simulink model "M182_Lab2"  (R2019b)
settings: Solver=ode45  StartTime=0.0  StopTime=10  RelTol=1e-5
settings Model: Creator=scjcb  LastModifiedBy=scjcb

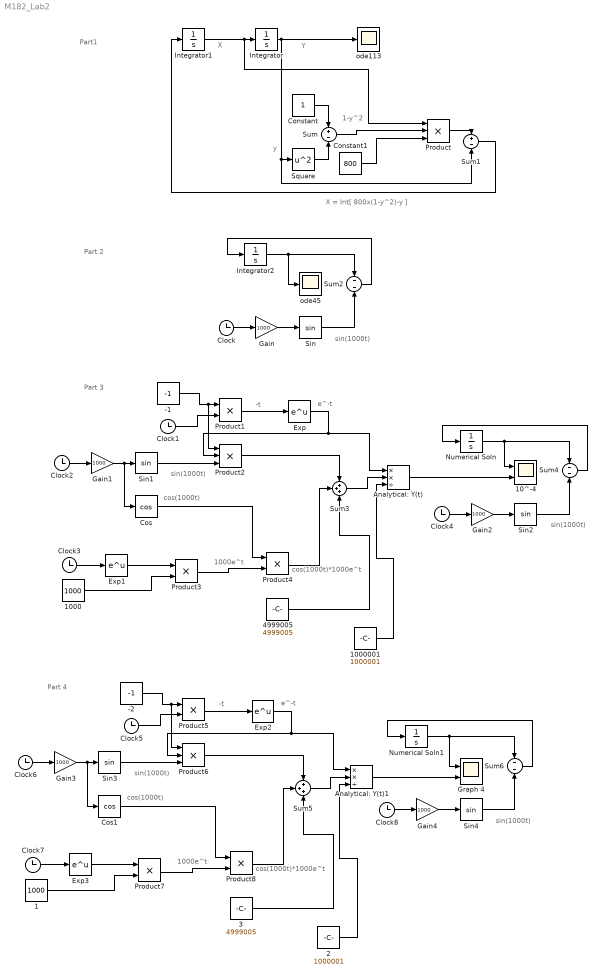
== system M182_Lab2 ==
  note: Part 3
  note: Part 2
  note: Part1
  note: cos(1000t)*1000e^t
  note: cos(1000t)
  note: 1000e^t
  note: e^-t
  note: -t
  note: sin(1000t)
  note: X
  note: Y
  note: X = Int[ 800x(1-y^2)-y ]
  note: 1-y^2
  note: y
  note: sin(1000t)
  note: sin(1000t)
  note: cos(1000t)*1000e^t
  note: e^-t
  note: 1000e^t
  note: Part 4
  note: sin(1000t)
  note: cos(1000t)
  note: sin(1000t)
  note: -t
  -1 : Constant  Value=-1
  -2 : Constant  Value=-1
  1 : Constant  Value=1000
  1000 : Constant  Value=1000
  1000001 : Constant  Value=1000001
  10^-4 : Scope  NumInputPorts=2
  2 : Constant  Value=1000001
  3 : Constant  Value=4999005
  4999005 : Constant  Value=4999005
  Analytical: Y(t) : Product  Inputs=**/
  Analytical: Y(t)1 : Product  Inputs=**/
  Clock{,1..8} (9 alike) : Clock
  Constant : Constant
  Constant1 : Constant  Value=800
  Cos : Trigonometry  Operator=cos
  Cos1 : Trigonometry  Operator=cos
  Exp{,1..3} (4 alike) : Math  SignedPower=off  SaturateOnIntegerOverflow=on
  Gain{,1..4} (5 alike) : Gain  Gain=1000
  Graph 4 : Scope  NumInputPorts=2
  Integrator : Integrator  InitialCondition=2
  Integrator1 : Integrator
  Integrator2 : Integrator  InitialCondition=5
  Numerical Soln : Integrator  InitialCondition=5
  Numerical Soln1 : Integrator  InitialCondition=5
  Product : Product  Inputs=3
  Product{1,3..5,7..8} (6 alike) : Product
  Product2 : Product  Inputs=3
  Product6 : Product  Inputs=3
  Sin{,1..4} (5 alike) : Trigonometry
  Square : Math  Operator=square  SignedPower=off  SaturateOnIntegerOverflow=on
  Sum : Sum  Inputs=+-
  Sum1 : Sum  Inputs=+-
  Sum2 : Sum  Inputs=--
  Sum3 : Sum  Inputs=+++
  Sum4 : Sum  Inputs=--
  Sum5 : Sum  Inputs=+++
  Sum6 : Sum  Inputs=--
  ode113 : Scope
  "ode45 " : Scope
  wires:
  Constant/1 -> Sum/1
  Integrator1/1 -> Product/1, Integrator/1
  Square/1 -> Sum/2
  Constant1/1 -> Product/3
  Sum/1 -> Product/2
  Product/1 -> Sum1/1
  Sum1/1 -> Integrator1/1
  Integrator/1 -> Sum1/2, Square/1, ode113/1
  Clock/1 -> Gain/1
  Gain/1 -> Sin/1
  Sin/1 -> Sum2/2
  Integrator2/1 -> "ode45 "/1, Sum2/1
  Sum2/1 -> Integrator2/1
  -1/1 -> Product2/1, Product1/1
  Clock1/1 -> Product1/2
  Product1/1 -> Exp/1
  Exp/1 -> Analytical: Y(t)/1, Product2/2
  Gain1/1 -> Cos/1, Sin1/1
  Clock2/1 -> Gain1/1
  Sin1/1 -> Product2/3
  Clock3/1 -> Exp1/1
  Exp1/1 -> Product3/1
  1000/1 -> Product3/2
  Cos/1 -> Product4/1
  Product3/1 -> Product4/2
  Product2/1 -> Sum3/1
  Product4/1 -> Sum3/2
  4999005/1 -> Sum3/3
  Sum3/1 -> Analytical: Y(t)/2
  1000001/1 -> Analytical: Y(t)/3
  Numerical Soln/1 -> 10^-4/1, Sum4/1
  Sin2/1 -> Sum4/2
  Clock4/1 -> Gain2/1
  Gain2/1 -> Sin2/1
  Sum4/1 -> Numerical Soln/1
  Analytical: Y(t)/1 -> 10^-4/2
  Exp3/1 -> Product7/1
  Clock5/1 -> Product5/2
  Product8/1 -> Sum5/2
  Clock8/1 -> Gain4/1
  Numerical Soln1/1 -> Graph 4/1, Sum6/1
  Sin4/1 -> Sum6/2
  2/1 -> Analytical: Y(t)1/3
  Product6/1 -> Sum5/1
  Sin3/1 -> Product6/3
  Exp2/1 -> Analytical: Y(t)1/1, Product6/2
  Clock6/1 -> Gain3/1
  Clock7/1 -> Exp3/1
  -2/1 -> Product6/1, Product5/1
  Sum5/1 -> Analytical: Y(t)1/2
  1/1 -> Product7/2
  Gain4/1 -> Sin4/1
  Sum6/1 -> Numerical Soln1/1
  3/1 -> Sum5/3
  Gain3/1 -> Cos1/1, Sin3/1
  Product5/1 -> Exp2/1
  Cos1/1 -> Product8/1
  Product7/1 -> Product8/2
  Analytical: Y(t)1/1 -> Graph 4/2
